simulink model "Lab1_Exercise_4_simulink"  (R2024a)
settings: Solver=VariableStepAuto  StartTime=0.0  StopTime=5  FixedStep=1  RelTol=1e-3
settings Model: Creator=Hp  LastModifiedBy=Hp

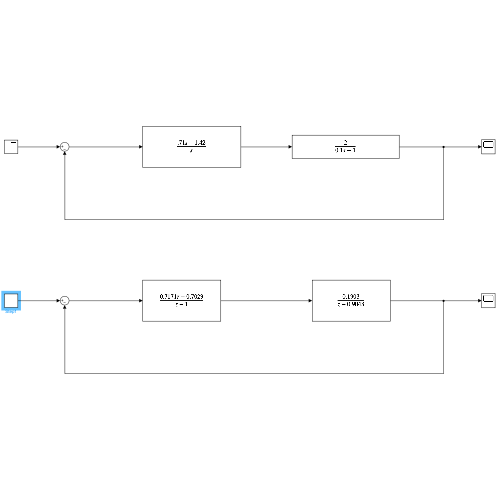
[thumbnail: Simulink's stored preview of the top-level diagram]
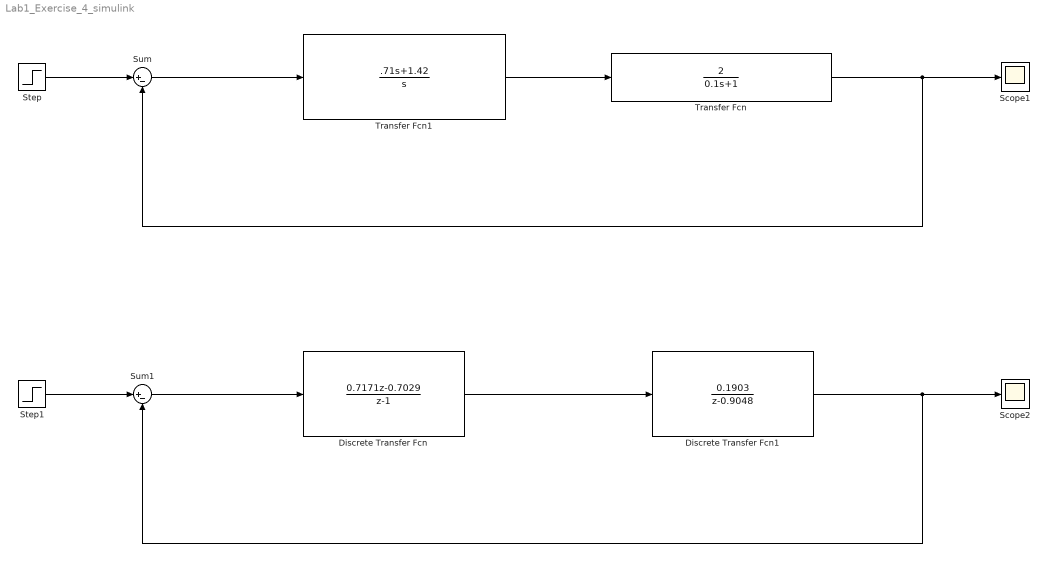
== system Lab1_Exercise_4_simulink ==
  Discrete Transfer Fcn : DiscreteTransferFcn  Numerator=[0.7171 -0.7029]  Denominator=[1 -1]
  Discrete Transfer Fcn1 : DiscreteTransferFcn  Numerator=[0.1903]  Denominator=[1 -0.9048]
  Scope1 : Scope
  Scope2 : Scope
  Step : Step  SampleTime=0.01
  Step1 : Step  SampleTime=0.01
  Sum : Sum  Inputs=|+-
  Sum1 : Sum  Inputs=|+-
  Transfer Fcn : TransferFcn  Numerator=[2]  Denominator=[0.1 1]
  Transfer Fcn1 : TransferFcn  Numerator=[.71 1.42]  Denominator=[1 0]
  wires:
  Step/1 -> Sum/1
  Transfer Fcn/1 -> Sum/2, Scope1/1
  Sum/1 -> Transfer Fcn1/1
  Transfer Fcn1/1 -> Transfer Fcn/1
  Discrete Transfer Fcn1/1 -> Sum1/2, Scope2/1
  Step1/1 -> Sum1/1
  Sum1/1 -> Discrete Transfer Fcn/1
  Discrete Transfer Fcn/1 -> Discrete Transfer Fcn1/1
